simulink model "simulink_caso4_adc"  (R2023a)
settings: Solver=VariableStepAuto  StartTime=0.0  StopTime=5  RelTol=1e-3
undefined symbols (not defined in the file): A, Aestd, B, Bestd, C, Cestd, D, Destd, K00d, Kd, Ts
libraries: simulink x1
settings Model: Creator=Agustin  LastModifiedBy=Agustin

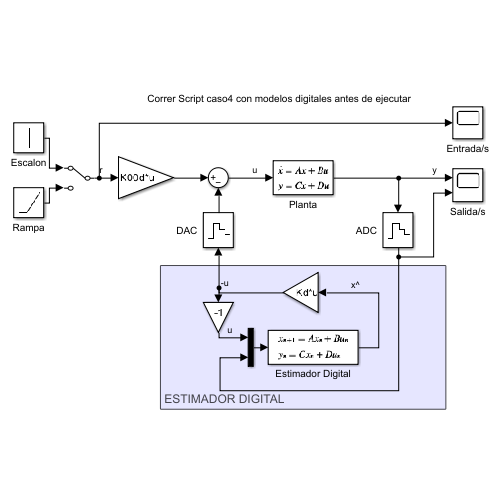
[thumbnail: Simulink's stored preview of the top-level diagram]
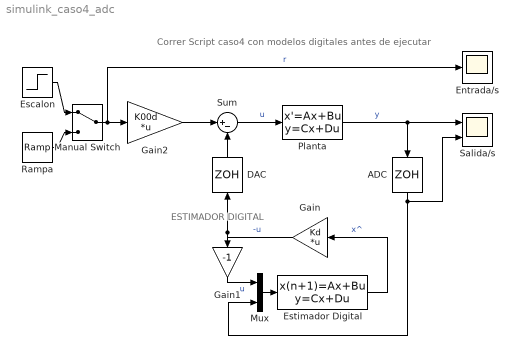
== system simulink_caso4_adc ==
  note: ESTIMADOR DIGITAL
  note: Correr Script caso4 con modelos digitales antes de ejecutar
  ADC : ZeroOrderHold  SampleTime=Ts
  DAC : ZeroOrderHold  SampleTime=Ts
  Entrada/s : Scope
  Escalon : Step  Time=0  SampleTime=0
  Estimador Digital : DiscreteStateSpace  A=Aestd  B=Bestd  C=Cestd  D=Destd  SampleTime=Ts
  Gain : Gain  Gain=Kd  Multiplication=Matrix(K*u)
  Gain1 : Gain  Gain=-1
  Gain2 : Gain  Gain=K00d  Multiplication=Matrix(K*u)
  Manual Switch : ManualSwitch
  Mux : Mux  Inputs=2
  Planta : StateSpace  A=A  B=B  C=C  D=D  InitialCondition=0
  Rampa : simulink/Sources/Ramp  slope=1  start=0  InitialOutput=0
  Salida/s : Scope  NumInputPorts=2
  Sum : Sum  Inputs=|+-
  wires:
  Sum/1 -> Planta/1  "u"
  Planta/1 -> ADC/1, Salida/s/1  "y"
  Manual Switch/1 -> Entrada/s/1, Gain2/1  "r"
  Gain/1 -> DAC/1, Gain1/1  "-u"
  Gain2/1 -> Sum/1
  Gain1/1 -> Mux/1  "u"
  Escalon/1 -> Manual Switch/1
  Rampa/1 -> Manual Switch/2
  DAC/1 -> Sum/2
  ADC/1 -> Mux/2, Salida/s/2
  Mux/1 -> Estimador Digital/1
  Estimador Digital/1 -> Gain/1  "x^"
